simulink model "Comprobar_Posicion_PID_ISA"  (R2021b)
settings: Solver=ode45  StartTime=0.0  StopTime=100  RelTol=1e-3  EnableMultiTasking=on
undefined symbols (not defined in the file or in its folder): airspeed_0, alpha_0, altitude_0, beta_0, deflect_sat, Earth, euler_0, h0, JSBSim, local_V_0, mTotal, Pos_0, pqr_0, r_MotorLeft, r_MotorRight, theta_0, Vel_0, VTOL_FW, WGS84
libraries: simulink_need_slupdate x5, aerolibfltsims x4, sharedutil x3, sharedtransform x2, aerolibtransform2 x1, aerolibutil x1
(part 1 of 2)
settings Model: Creator=Fede Paredes  LastModifiedBy=Jose Luis Musoles
settings SolverCC: AlgebraicLoopSolver=TrustRegion
settings DataIOCC: LimitDataPoints=on  SaveFormat=Array  ReturnWorkspaceOutputs=off
settings OptimizationCC: LifeSpan=inf
settings DebuggingCC: UnderspecifiedInitializationDetection=Classic  MergeDetectMultiDrivingBlocksExec=none  SolverPrmCheckMsg=warning  StateNameClashWarn=warning  SFUnexpectedBacktrackingDiag=warning  SFNoUnconditionalDefaultTransitionDiag=warning  SFExecutionAtInitializationDiag=none  SFMachineParentedDataDiag=warning  ArithmeticOperatorsInVariantConditions=warning
settings HardwareCC: ProdBitPerPointer=32  ProdBitPerSizeT=32  ProdBitPerPtrDiffT=32  ProdLargestAtomicFloat=None  ProdIntDivRoundTo=Undefined  ProdEndianess=Unspecified  ProdWordSize=32  ProdHWDeviceType=32-bit Generic
settings ModelReferenceCC: PropagateSignalLabelsOutOfModel=off
settings SFSimCC: SimUseLocalCustomCode=off  CustomCodeUndefinedFunction=UseInterfaceOnly
settings RTWCC: RTWUseLocalCustomCode=off
settings CodeAppCC: StateflowObjectComments=on
settings GRTTargetCC: TargetLangStandard=C89/C90 (ANSI)
settings ConfigComp: CovMetricSettings=dw  CovSaveCumulativeToWorkspaceVar=on  CovSaveSingleToWorkspaceVar=on  CovExternalEMLEnable=off

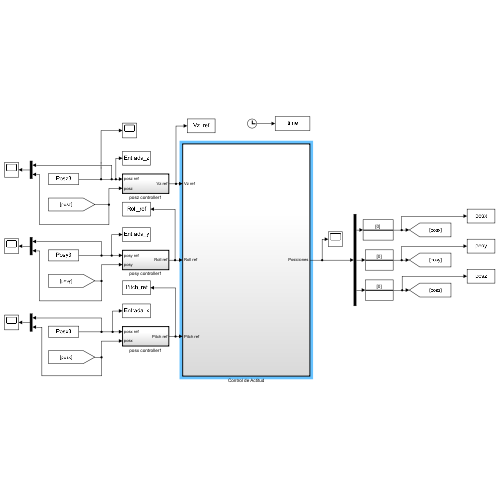
[thumbnail: Simulink's stored preview of the top-level diagram]
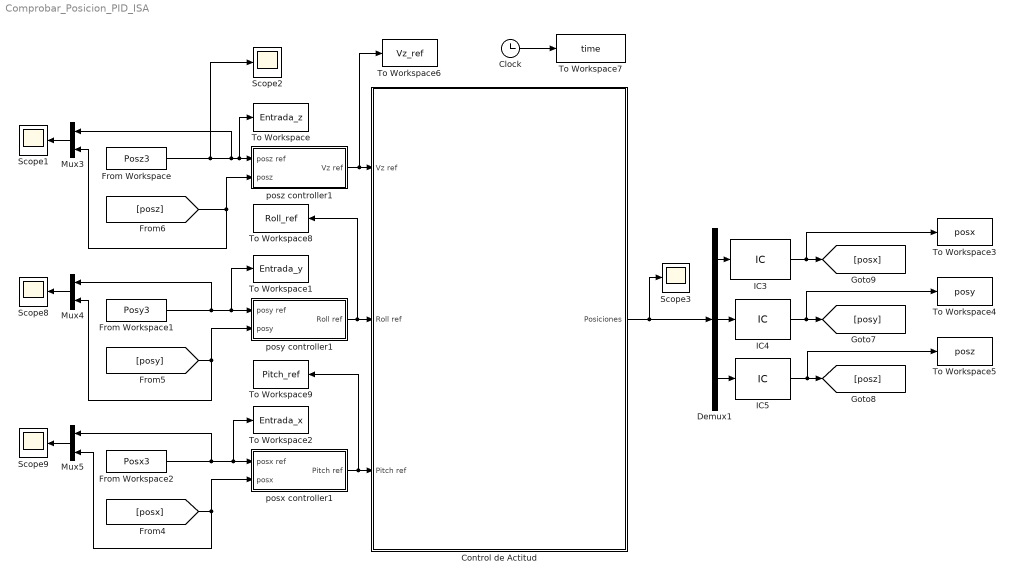
== system Comprobar_Posicion_PID_ISA ==
  Clock : Clock
  Control de Actitud : Subsystem  TreatAsAtomicUnit=on
  Demux1 : Demux  Outputs=3
  From Workspace : FromWorkspace  VariableName=Posz3
  From Workspace1 : FromWorkspace  VariableName=Posy3
  From Workspace2 : FromWorkspace  VariableName=Posx3
  IC3 : InitialCondition  Value=0
  IC4 : InitialCondition  Value=0
  IC5 : InitialCondition  Value=0
  Mux3 : Mux  Inputs=2
  Mux4 : Mux  Inputs=2
  Mux5 : Mux  Inputs=2
  Scope{1..3,8..9} (5 alike) : Scope
  To Workspace : ToWorkspace  VariableName=Entrada_z  SaveFormat=Timeseries  SampleTime=-1
  To Workspace1 : ToWorkspace  VariableName=Entrada_y  SaveFormat=Timeseries  SampleTime=-1
  To Workspace2 : ToWorkspace  VariableName=Entrada_x  SaveFormat=Timeseries  SampleTime=-1
  To Workspace3 : ToWorkspace  VariableName=posx  SaveFormat=Timeseries  SampleTime=-1
  To Workspace4 : ToWorkspace  VariableName=posy  SaveFormat=Timeseries  SampleTime=-1
  To Workspace5 : ToWorkspace  VariableName=posz  SaveFormat=Timeseries  SampleTime=-1
  To Workspace6 : ToWorkspace  VariableName=Vz_ref  SaveFormat=Timeseries  SampleTime=-1
  To Workspace7 : ToWorkspace  VariableName=time  SaveFormat=Timeseries  SampleTime=-1
  To Workspace8 : ToWorkspace  VariableName=Roll_ref  SaveFormat=Timeseries  SampleTime=-1
  To Workspace9 : ToWorkspace  VariableName=Pitch_ref  SaveFormat=Timeseries  SampleTime=-1
  posx controller1 : Subsystem  TreatAsAtomicUnit=on
  posy controller1 : Subsystem  TreatAsAtomicUnit=on
  posz controller1 : Subsystem  TreatAsAtomicUnit=on
  wires:
  Control de Actitud/1(Posiciones) -> Demux1/1, Scope3/1
  Demux1/1 -> IC3/1
  Demux1/2 -> IC4/1
  Demux1/3 -> IC5/1
  posy controller1/1(Roll ref) -> To Workspace8/1, Control de Actitud/2(Roll ref)
  posx controller1/1(Pitch ref) -> To Workspace9/1, Control de Actitud/3(Pitch ref)
  [posx] -> posx controller1/2(posx), Mux5/2
  [posz] -> posz controller1/2(posz), Mux3/2
  [posy] -> posy controller1/2(posy), Mux4/2
  Mux3/1 -> Scope1/1
  Mux4/1 -> Scope8/1
  Mux5/1 -> Scope9/1
  From Workspace1/1 -> To Workspace1/1, posy controller1/1(posy ref), Mux4/1
  From Workspace2/1 -> To Workspace2/1, posx controller1/1(posx ref), Mux5/1
  From Workspace/1 -> Scope2/1, Mux3/1, To Workspace/1, posz controller1/1(posz ref)
  Clock/1 -> To Workspace7/1
  posz controller1/1(Vz ref) -> To Workspace6/1, Control de Actitud/1(Vz ref)
  IC5/1 -> To Workspace5/1, [posz]
  IC3/1 -> To Workspace3/1, [posx]
  IC4/1 -> To Workspace4/1, [posy]

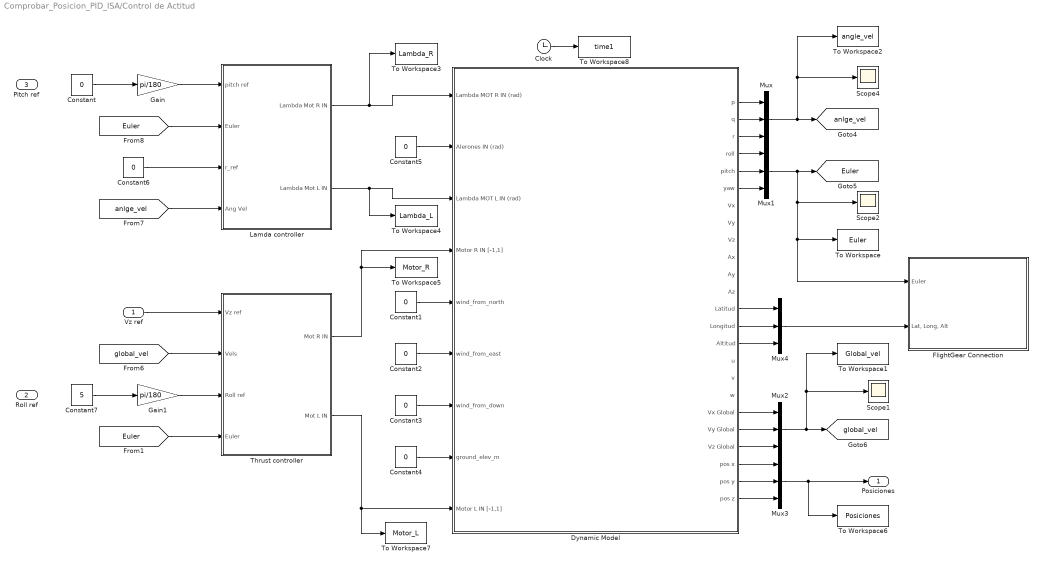
== system Comprobar_Posicion_PID_ISA/Control de Actitud ==
  Vz ref : Inport
  Roll ref : Inport  Port=2
  Pitch ref : Inport  Port=3
  Clock : Clock
  Constant{,1..6} (7 alike) : Constant  Value=0
  Constant7 : Constant  Value=5
  Dynamic Model : Subsystem  TreatAsAtomicUnit=on
  FlightGear Connection : Subsystem  TreatAsAtomicUnit=on
  Gain : Gain  Gain=pi/180
  Gain1 : Gain  Gain=pi/180
  Lamda controller : Subsystem
  Mux{,1..4} (5 alike) : Mux  Inputs=3
  Scope1 : Scope
  Scope2 : Scope
  Scope4 : Scope
  Thrust controller : Subsystem
  To Workspace : ToWorkspace  VariableName=Euler  SaveFormat=Timeseries  SampleTime=-1
  To Workspace1 : ToWorkspace  VariableName=Global_vel  SaveFormat=Timeseries  SampleTime=-1
  To Workspace2 : ToWorkspace  VariableName=angle_vel  SaveFormat=Timeseries  SampleTime=-1
  To Workspace3 : ToWorkspace  VariableName=Lambda_R  SaveFormat=Timeseries  SampleTime=-1
  To Workspace4 : ToWorkspace  VariableName=Lambda_L  SaveFormat=Timeseries  SampleTime=-1
  To Workspace5 : ToWorkspace  VariableName=Motor_R  SaveFormat=Timeseries  SampleTime=-1
  To Workspace6 : ToWorkspace  VariableName=Posiciones  SaveFormat=Timeseries  SampleTime=-1
  To Workspace7 : ToWorkspace  VariableName=Motor_L  SaveFormat=Timeseries  SampleTime=-1
  To Workspace8 : ToWorkspace  VariableName=time1  SaveFormat=Timeseries  SampleTime=-1
  Posiciones : Outport
  tag scope: Euler=global, anlge_vel=global, global_vel=global
  wires:
  Dynamic Model/1(p) -> Mux/1
  Dynamic Model/3(r) -> Mux/3
  Mux/1 -> To Workspace2/1, Scope4/1, [anlge_vel]
  Dynamic Model/4(roll) -> Mux1/1
  Dynamic Model/6(yaw) -> Mux1/3
  Mux1/1 -> FlightGear Connection/1("Euler "), To Workspace/1, Scope2/1, [Euler]
  Dynamic Model/2(q) -> Mux/2
  Dynamic Model/5(pitch) -> Mux1/2
  Mux2/1 -> Scope1/1, To Workspace1/1, [global_vel]
  [global_vel] -> Thrust controller/2(Vels)
  Thrust controller/1(Mot R IN) -> To Workspace5/1, Dynamic Model/4(Motor R IN [-1,1])
  Thrust controller/2(Mot L IN) -> To Workspace7/1, Dynamic Model/9(Motor L IN [-1,1])
  [Euler] -> Thrust controller/4(Euler)
  [Euler] -> Lamda controller/2(Euler)
  [anlge_vel] -> Lamda controller/4(Ang Vel)
  Lamda controller/1(Lambda Mot R IN) -> To Workspace3/1, Dynamic Model/1(Lambda MOT R IN (rad))
  Lamda controller/2(Lambda Mot L IN) -> To Workspace4/1, Dynamic Model/3(" Lambda MOT L IN (rad)")
  Constant5/1 -> Dynamic Model/2(Alerones IN (rad))
  Vz ref/1 -> Thrust controller/1(Vz ref)
  Constant6/1 -> Lamda controller/3(r_ref)
  Mux3/1 -> Posiciones/1, To Workspace6/1
  Constant1/1 -> Dynamic Model/5(wind_from_north)
  Constant2/1 -> Dynamic Model/6(wind_from_east)
  Constant3/1 -> Dynamic Model/7(wind_from_down)
  Constant4/1 -> Dynamic Model/8(ground_elev_m)
  Dynamic Model/22(pos x) -> Mux3/1
  Dynamic Model/23(pos y) -> Mux3/2
  Dynamic Model/24(pos z) -> Mux3/3
  Dynamic Model/19(Vx Global) -> Mux2/1
  Dynamic Model/20(Vy Global) -> Mux2/2
  Dynamic Model/21(Vz Global) -> Mux2/3
  Clock/1 -> To Workspace8/1
  Dynamic Model/13(Latitud) -> Mux4/1
  Dynamic Model/14(Longitud) -> Mux4/2
  Dynamic Model/15(Altitud) -> Mux4/3
  Mux4/1 -> FlightGear Connection/2("Lat, Long, Alt ")
  Constant/1 -> Gain/1
  Gain/1 -> Lamda controller/1(pitch ref)
  Constant7/1 -> Gain1/1
  Gain1/1 -> Thrust controller/3(Roll ref)

== system Comprobar_Posicion_PID_ISA/posx controller1 ==
  posx ref : Inport
  posx : Inport  Port=2
  Constant : Constant  Value=0
  PID ISA : Subsystem  mask{kc=-0.5363, Ti=17.0146, Td=0.8299}
  Rate Transition : RateTransition  OutPortSampleTime=2e-2
  Rate Transition1 : RateTransition  OutPortSampleTime=2e-2
  Scope4 : Scope
  Pitch ref : Outport
  wires:
  posx ref/1 -> Rate Transition/1
  posx/1 -> Rate Transition1/1
  Constant/1 -> PID ISA/3(u0)
  Rate Transition/1 -> PID ISA/1(Reference)
  Rate Transition1/1 -> PID ISA/2(Vc)
  PID ISA/1(Vm) -> Scope4/1, Pitch ref/1

== system Comprobar_Posicion_PID_ISA/posy controller1 ==
  posy ref : Inport
  posy : Inport  Port=2
  Constant : Constant  Value=0
  PID ISA : Subsystem  mask{kc=0.5691, Ti=16.6404, Td=0.9487}
  Rate Transition : RateTransition  OutPortSampleTime=2e-2
  Rate Transition1 : RateTransition  OutPortSampleTime=2e-2
  Scope4 : Scope
  Roll ref : Outport
  wires:
  Constant/1 -> PID ISA/3(u0)
  posy ref/1 -> Rate Transition/1
  Rate Transition/1 -> PID ISA/1(Reference)
  posy/1 -> Rate Transition1/1
  Rate Transition1/1 -> PID ISA/2(Vc)
  PID ISA/1(Vm) -> Scope4/1, Roll ref/1

== system Comprobar_Posicion_PID_ISA/posz controller1 ==
  note: Se ha modificado la derivada
  posz ref : Inport
  posz : Inport  Port=2
  Constant : Constant  Value=0
  PID ISA : Subsystem  mask{kc=0.9270, Ti=10.0761, Td=0.4708}
  Rate Transition : RateTransition  OutPortSampleTime=2e-2
  Rate Transition1 : RateTransition  OutPortSampleTime=2e-2
  Scope4 : Scope
  Vz ref : Outport
  wires:
  Constant/1 -> PID ISA/3(u0)
  posz ref/1 -> Rate Transition/1
  Rate Transition/1 -> PID ISA/1(Reference)
  posz/1 -> Rate Transition1/1
  Rate Transition1/1 -> PID ISA/2(Vc)
  PID ISA/1(Vm) -> Scope4/1, Vz ref/1

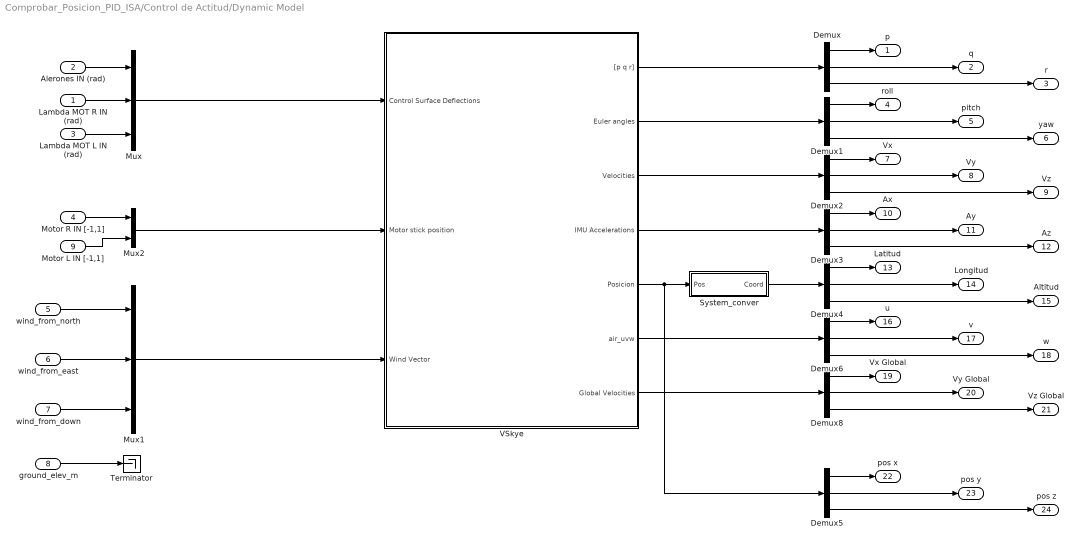
== system Comprobar_Posicion_PID_ISA/Control de Actitud/Dynamic Model ==
  Lambda MOT R IN (rad) : Inport
  Alerones IN (rad) : Inport  Port=2
  " Lambda MOT L IN (rad)" : Inport  Port=3
  Motor R IN [-1,1] : Inport  Port=4
  wind_from_north : Inport  Port=5
  wind_from_east : Inport  Port=6
  wind_from_down : Inport  Port=7
  ground_elev_m : Inport  Port=8
  Motor L IN [-1,1] : Inport  Port=9
  Demux{,1..6,8} (8 alike) : Demux  Outputs=3
  Mux : Mux  Inputs=3
  Mux1 : Mux  Inputs=3
  Mux2 : Mux  Inputs=2
  System_conver : Subsystem
  Terminator : Terminator
  VSkye : Subsystem
  p : Outport
  q : Outport  Port=2
  r : Outport  Port=3
  roll : Outport  Port=4
  pitch : Outport  Port=5
  yaw : Outport  Port=6
  Vx : Outport  Port=7
  Vy : Outport  Port=8
  Vz : Outport  Port=9
  Ax : Outport  Port=10
  Ay : Outport  Port=11
  Az : Outport  Port=12
  Latitud : Outport  Port=13
  Longitud : Outport  Port=14
  Altitud : Outport  Port=15
  u : Outport  Port=16
  v : Outport  Port=17
  w : Outport  Port=18
  Vx Global : Outport  Port=19
  Vy Global : Outport  Port=20
  Vz Global : Outport  Port=21
  pos x : Outport  Port=22
  pos y : Outport  Port=23
  pos z : Outport  Port=24
  wires:
  VSkye/2(Euler angles) -> Demux1/1
  VSkye/3(Velocities) -> Demux2/1
  Mux1/1 -> VSkye/3(Wind Vector)
  VSkye/5(Posicion) -> Demux5/1, System_conver/1(Pos)
  Mux/1 -> VSkye/1(Control Surface Deflections)
  VSkye/4("IMU Accelerations ") -> Demux3/1
  VSkye/1("[p q r]") -> Demux/1
  Alerones IN (rad)/1 -> Mux/1
  Lambda MOT R IN (rad)/1 -> Mux/2
  " Lambda MOT L IN (rad)"/1 -> Mux/3
  Demux/1 -> p/1
  Demux/2 -> q/1
  Demux/3 -> r/1
  Demux1/1 -> roll/1
  Demux1/2 -> pitch/1
  Demux1/3 -> yaw/1
  Demux2/1 -> Vx/1
  Demux2/2 -> Vy/1
  Demux2/3 -> Vz/1
  Demux3/1 -> Ax/1
  Demux3/2 -> Ay/1
  Demux3/3 -> Az/1
  Demux4/1 -> Latitud/1
  Demux4/2 -> Longitud/1
  Demux4/3 -> Altitud/1
  Demux6/1 -> u/1
  Demux6/2 -> v/1
  Demux6/3 -> w/1
  Demux5/1 -> pos x/1
  Demux5/2 -> pos y/1
  Demux5/3 -> pos z/1
  VSkye/6(air_uvw) -> Demux6/1
  System_conver/1(Coord) -> Demux4/1
  wind_from_north/1 -> Mux1/1
  wind_from_east/1 -> Mux1/2
  wind_from_down/1 -> Mux1/3
  Motor R IN [-1,1]/1 -> Mux2/1
  Mux2/1 -> VSkye/2(Motor stick position)
  Motor L IN [-1,1]/1 -> Mux2/2
  ground_elev_m/1 -> Terminator/1
  Demux8/1 -> Vx Global/1
  Demux8/2 -> Vy Global/1
  Demux8/3 -> Vz Global/1
  VSkye/7(Global Velocities) -> Demux8/1

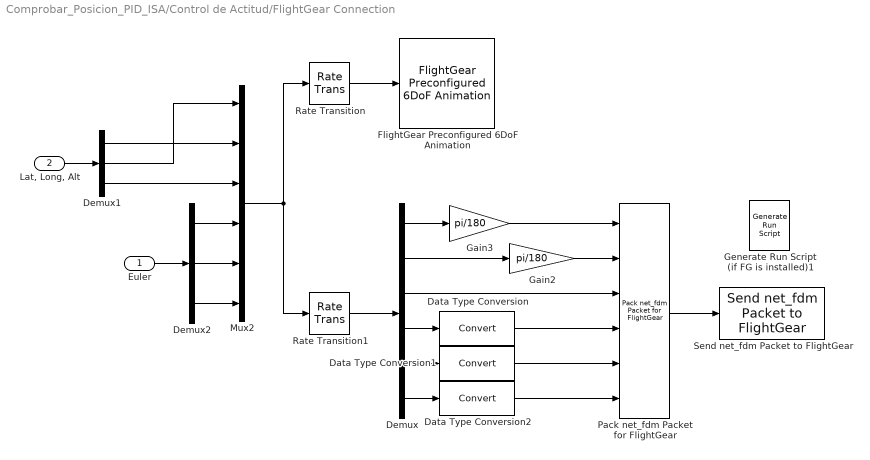
== system Comprobar_Posicion_PID_ISA/Control de Actitud/FlightGear Connection ==
  "Euler " : Inport
  "Lat, Long, Alt " : Inport  Port=2
  Data Type Conversion : DataTypeConversion  SampleTime=0.01
  Data Type Conversion1 : DataTypeConversion  SampleTime=0.01
  Data Type Conversion2 : DataTypeConversion  SampleTime=0.01
  Demux : Demux  Outputs=6
  Demux1 : Demux  Outputs=3
  Demux2 : Demux  Outputs=3
  FlightGear Preconfigured 6DoF Animation : aerolibfltsims/FlightGear Preconfigured 6DoF Animation  xFlightGearVersion=v2.6  DestinationIpAddress=127.0.0.1  DestinationPort=5502  SampleTime=0.01  packetVersion=24
  Gain2 : Gain  Gain=pi/180
  Gain3 : Gain  Gain=pi/180
  Generate Run Script (if FG is installed)1 : aerolibfltsims/Generate Run Script  Architecture=Default  dataFlow=Send  GeometryModelName=VTOL_FW-JSBSim  AirportId=KSFO  RunwayId=10L  InitialAltitude=7224  InitialHeading=113  OffsetDistance=4.72  OffsetAzimuth=0  InstallScenery=off  DisableShaders=off  OriginAddress=127.0.0.1  DestinationPort=5502  OriginPort=5505  LocalAddress=127.0.0.1  OutputFileName=FW_Simulink26.bat  FlightGearBaseDirectory=C:\Program Files\FlightGear2.6
  Mux2 : Mux  Inputs=6
  Pack net_fdm Packet for FlightGear : aerolibfltsims/Pack net_fdm Packet for FlightGear  FlightGearVersion=v2.6  ShowPositionAttitudeInputs=on  ShowVelocityAccelerationInputs=off  ShowControlSurfacePositionInputs=off  ShowEngineFuelInputs=off  ShowLandingGearInputs=off  ShowEnvironmentInputs=off  SampleTime=0.01  packetVersion=24
      settings: SourceProductBaseCode=AE
  Rate Transition : RateTransition  InitialCondition=[0,0,0,pi,0,0]
  Rate Transition1 : RateTransition  InitialCondition=[0,0,0,0,0,0]
  Send net_fdm Packet to FlightGear : aerolibfltsims/Send net_fdm Packet to FlightGear  DestinationIpAddress=127.0.0.1  DestinationPort=5502  LocalIpPort=-1  varLen=off  SampleTime=0.01
      settings: SourceProductBaseCode=AE
  wires:
  Demux2/1 -> Mux2/4
  Demux2/2 -> Mux2/5
  Demux2/3 -> Mux2/6
  Demux/1 -> Gain3/1
  Demux/2 -> Gain2/1
  Demux/3 -> Pack net_fdm Packet for FlightGear/3
  Pack net_fdm Packet for FlightGear/1 -> Send net_fdm Packet to FlightGear/1
  "Euler "/1 -> Demux2/1
  "Lat, Long, Alt "/1 -> Demux1/1
  Rate Transition/1 -> FlightGear Preconfigured 6DoF Animation/1
  Rate Transition1/1 -> Demux/1
  Demux/6 -> Data Type Conversion2/1
  Demux/5 -> Data Type Conversion1/1
  Demux/4 -> Data Type Conversion/1
  Data Type Conversion/1 -> Pack net_fdm Packet for FlightGear/4
  Data Type Conversion1/1 -> Pack net_fdm Packet for FlightGear/5
  Data Type Conversion2/1 -> Pack net_fdm Packet for FlightGear/6
  Demux1/3 -> Mux2/3
  Mux2/1 -> Rate Transition1/1, Rate Transition/1
  Gain3/1 -> Pack net_fdm Packet for FlightGear/1
  Gain2/1 -> Pack net_fdm Packet for FlightGear/2
  Demux1/1 -> Mux2/2
  Demux1/2 -> Mux2/1

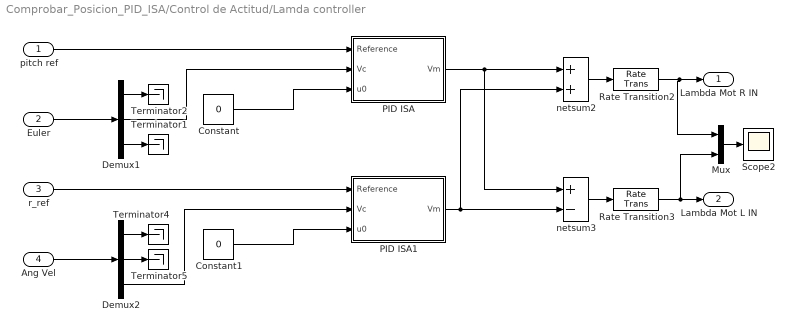
== system Comprobar_Posicion_PID_ISA/Control de Actitud/Lamda controller ==
  pitch ref : Inport
  Euler : Inport  Port=2
  r_ref : Inport  Port=3
  Ang Vel : Inport  Port=4
  Constant : Constant  Value=0
  Constant1 : Constant  Value=0
  Demux1 : Demux  Outputs=3
  Demux2 : Demux  Outputs=3
  Mux : Mux  Inputs=2
  PID ISA : Subsystem  mask{kc=0.549, Ti=0.450, Td=0.111}
  PID ISA1 : Subsystem  mask{kc=0.2421, Ti=6.3879, Td=0.0264}
  Rate Transition2 : RateTransition  OutPortSampleTime=1e-2
  Rate Transition3 : RateTransition  OutPortSampleTime=1e-2
  Scope2 : Scope
  Terminator{1..2,4..5} (4 alike) : Terminator
  netsum2 : Sum  Inputs=2  InputSameDT=on  SaturateOnIntegerOverflow=on  OutDataTypeStr=Inherit: Same as first input
  netsum3 : Sum  Inputs=+-  InputSameDT=on  SaturateOnIntegerOverflow=on  OutDataTypeStr=Inherit: Same as first input
  Lambda Mot R IN : Outport
  Lambda Mot L IN : Outport  Port=2
  wires:
  Demux1/1 -> Terminator2/1
  Euler/1 -> Demux1/1
  Demux1/3 -> Terminator1/1
  Demux2/1 -> Terminator4/1
  Ang Vel/1 -> Demux2/1
  Demux2/2 -> Terminator5/1
  PID ISA/1(Vm) -> netsum3/1, netsum2/1
  PID ISA1/1(Vm) -> netsum2/2, netsum3/2
  netsum2/1 -> Rate Transition2/1
  netsum3/1 -> Rate Transition3/1
  pitch ref/1 -> PID ISA/1(Reference)
  r_ref/1 -> PID ISA1/1(Reference)
  Demux1/2 -> PID ISA/2(Vc)
  Constant/1 -> PID ISA/3(u0)
  Demux2/3 -> PID ISA1/2(Vc)
  Constant1/1 -> PID ISA1/3(u0)
  Rate Transition2/1 -> Mux/1, Lambda Mot R IN/1
  Rate Transition3/1 -> Mux/2, Lambda Mot L IN/1
  Mux/1 -> Scope2/1

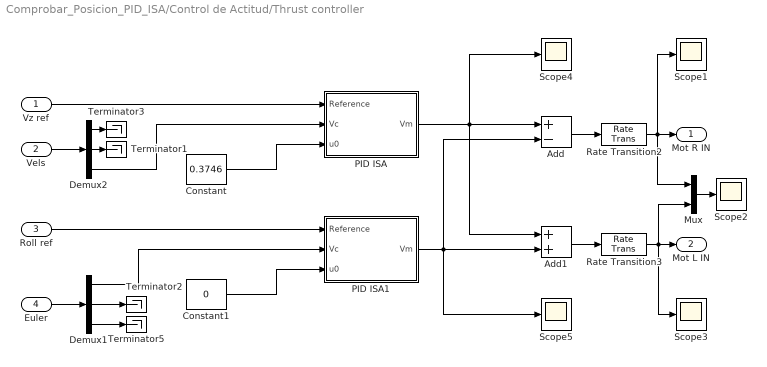
== system Comprobar_Posicion_PID_ISA/Control de Actitud/Thrust controller ==
  Vz ref : Inport
  Vels : Inport  Port=2
  Roll ref : Inport  Port=3
  Euler : Inport  Port=4
  Add : Sum  Inputs=+-
  Add1 : Sum
  Constant : Constant  Value=0.3746
  Constant1 : Constant  Value=0
  Demux1 : Demux  Outputs=3
  Demux2 : Demux  Outputs=3
  Mux : Mux  Inputs=2
  PID ISA : Subsystem  mask{kc=-0.42, Ti=11.3514, Td=0.0471}
  PID ISA1 : Subsystem  mask{kc=0.8757, Ti=0.4816, Td=0.1199}
  Rate Transition2 : RateTransition  OutPortSampleTime=1e-2
  Rate Transition3 : RateTransition  OutPortSampleTime=1e-2
  Scope{1..5} (5 alike) : Scope
  Terminator{1..3,5} (4 alike) : Terminator
  Mot R IN : Outport
  Mot L IN : Outport  Port=2
  wires:
  Mux/1 -> Scope2/1
  Constant1/1 -> PID ISA1/3(u0)
  Demux1/1 -> PID ISA1/2(Vc)
  Constant/1 -> PID ISA/3(u0)
  Demux2/3 -> PID ISA/2(Vc)
  Rate Transition3/1 -> Scope3/1, Mot L IN/1, Mux/2
  Rate Transition2/1 -> Mux/1, Scope1/1, Mot R IN/1
  Roll ref/1 -> PID ISA1/1(Reference)
  Vz ref/1 -> PID ISA/1(Reference)
  PID ISA1/1(Vm) -> Scope5/1, Add/2, Add1/2
  Add1/1 -> Rate Transition3/1
  PID ISA/1(Vm) -> Scope4/1, Add/1, Add1/1
  Add/1 -> Rate Transition2/1
  Demux1/3 -> Terminator5/1
  Demux1/2 -> Terminator2/1
  Euler/1 -> Demux1/1
  Vels/1 -> Demux2/1
  Demux2/2 -> Terminator1/1
  Demux2/1 -> Terminator3/1

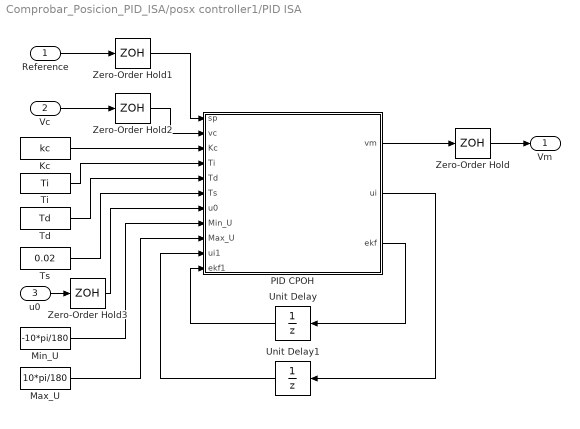
== system Comprobar_Posicion_PID_ISA/posx controller1/PID ISA ==
  Reference : Inport
  Vc : Inport  Port=2
  u0 : Inport  Port=3
  Kc : Constant  Value=kc
  Max_U : Constant  Value=10*pi/180
  Min_U : Constant  Value=-10*pi/180
  PID CPOH : MATLAB Function  TreatAsAtomicUnit=on
  Td : Constant  Value=Td
  Ti : Constant  Value=Ti
  Ts : Constant  Value=0.02
  Unit Delay : UnitDelay  SampleTime=0.02  HasFrameUpgradeWarning=on
  Unit Delay1 : UnitDelay  SampleTime=0.02  HasFrameUpgradeWarning=on
  Zero-Order Hold : ZeroOrderHold  SampleTime=0.02
  Zero-Order Hold1 : ZeroOrderHold  SampleTime=0.02
  Zero-Order Hold2 : ZeroOrderHold  SampleTime=0.02
  Zero-Order Hold3 : ZeroOrderHold  SampleTime=0.04
  Vm : Outport
  wires:
  Kc/1 -> PID CPOH/3(Kc)
  Ti/1 -> PID CPOH/4(Ti)
  Td/1 -> PID CPOH/5(Td)
  Ts/1 -> PID CPOH/6(Ts)
  u0/1 -> Zero-Order Hold3/1
  Min_U/1 -> PID CPOH/8(Min_U)
  Max_U/1 -> PID CPOH/9(Max_U)
  Unit Delay/1 -> PID CPOH/11(ekf1)
  PID CPOH/3(ekf) -> Unit Delay/1
  Unit Delay1/1 -> PID CPOH/10(ui1)
  PID CPOH/2(ui) -> Unit Delay1/1
  Reference/1 -> Zero-Order Hold1/1
  Vc/1 -> Zero-Order Hold2/1
  PID CPOH/1(vm) -> Zero-Order Hold/1
  Zero-Order Hold/1 -> Vm/1
  Zero-Order Hold1/1 -> PID CPOH/1(sp)
  Zero-Order Hold3/1 -> PID CPOH/7(u0)
  Zero-Order Hold2/1 -> PID CPOH/2(vc)

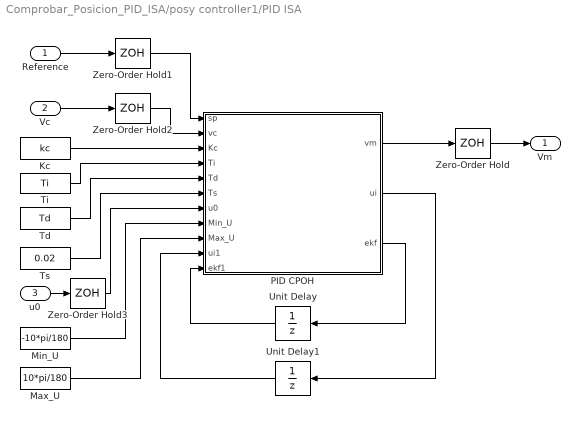
== system Comprobar_Posicion_PID_ISA/posy controller1/PID ISA ==
  Reference : Inport
  Vc : Inport  Port=2
  u0 : Inport  Port=3
  Kc : Constant  Value=kc
  Max_U : Constant  Value=10*pi/180
  Min_U : Constant  Value=-10*pi/180
  PID CPOH : MATLAB Function  TreatAsAtomicUnit=on
  Td : Constant  Value=Td
  Ti : Constant  Value=Ti
  Ts : Constant  Value=0.02
  Unit Delay : UnitDelay  SampleTime=0.02  HasFrameUpgradeWarning=on
  Unit Delay1 : UnitDelay  SampleTime=0.02  HasFrameUpgradeWarning=on
  Zero-Order Hold : ZeroOrderHold  SampleTime=0.02
  Zero-Order Hold1 : ZeroOrderHold  SampleTime=0.02
  Zero-Order Hold2 : ZeroOrderHold  SampleTime=0.02
  Zero-Order Hold3 : ZeroOrderHold  SampleTime=0.04
  Vm : Outport
  wires:
  Kc/1 -> PID CPOH/3(Kc)
  Ti/1 -> PID CPOH/4(Ti)
  Td/1 -> PID CPOH/5(Td)
  Ts/1 -> PID CPOH/6(Ts)
  u0/1 -> Zero-Order Hold3/1
  Min_U/1 -> PID CPOH/8(Min_U)
  Max_U/1 -> PID CPOH/9(Max_U)
  Unit Delay/1 -> PID CPOH/11(ekf1)
  PID CPOH/3(ekf) -> Unit Delay/1
  Unit Delay1/1 -> PID CPOH/10(ui1)
  PID CPOH/2(ui) -> Unit Delay1/1
  Reference/1 -> Zero-Order Hold1/1
  Vc/1 -> Zero-Order Hold2/1
  PID CPOH/1(vm) -> Zero-Order Hold/1
  Zero-Order Hold/1 -> Vm/1
  Zero-Order Hold1/1 -> PID CPOH/1(sp)
  Zero-Order Hold3/1 -> PID CPOH/7(u0)
  Zero-Order Hold2/1 -> PID CPOH/2(vc)

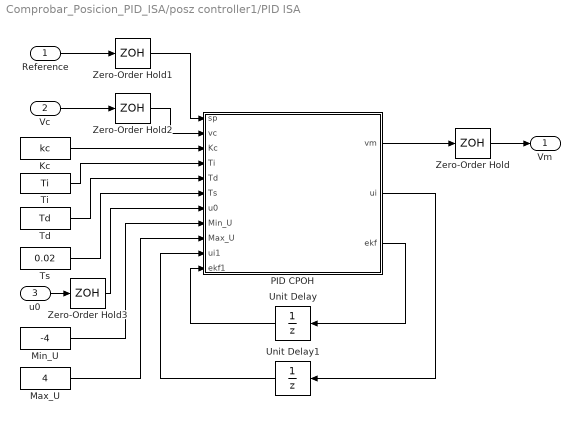
== system Comprobar_Posicion_PID_ISA/posz controller1/PID ISA ==
  Reference : Inport
  Vc : Inport  Port=2
  u0 : Inport  Port=3
  Kc : Constant  Value=kc
  Max_U : Constant  Value=4
  Min_U : Constant  Value=-4
  PID CPOH : MATLAB Function  TreatAsAtomicUnit=on
  Td : Constant  Value=Td
  Ti : Constant  Value=Ti
  Ts : Constant  Value=0.02
  Unit Delay : UnitDelay  SampleTime=0.02  HasFrameUpgradeWarning=on
  Unit Delay1 : UnitDelay  SampleTime=0.02  HasFrameUpgradeWarning=on
  Zero-Order Hold : ZeroOrderHold  SampleTime=0.02
  Zero-Order Hold1 : ZeroOrderHold  SampleTime=0.02
  Zero-Order Hold2 : ZeroOrderHold  SampleTime=0.02
  Zero-Order Hold3 : ZeroOrderHold  SampleTime=0.04
  Vm : Outport
  wires:
  Kc/1 -> PID CPOH/3(Kc)
  Ti/1 -> PID CPOH/4(Ti)
  Td/1 -> PID CPOH/5(Td)
  Ts/1 -> PID CPOH/6(Ts)
  u0/1 -> Zero-Order Hold3/1
  Min_U/1 -> PID CPOH/8(Min_U)
  Max_U/1 -> PID CPOH/9(Max_U)
  Unit Delay/1 -> PID CPOH/11(ekf1)
  PID CPOH/3(ekf) -> Unit Delay/1
  Unit Delay1/1 -> PID CPOH/10(ui1)
  PID CPOH/2(ui) -> Unit Delay1/1
  Reference/1 -> Zero-Order Hold1/1
  Vc/1 -> Zero-Order Hold2/1
  PID CPOH/1(vm) -> Zero-Order Hold/1
  Zero-Order Hold/1 -> Vm/1
  Zero-Order Hold1/1 -> PID CPOH/1(sp)
  Zero-Order Hold3/1 -> PID CPOH/7(u0)
  Zero-Order Hold2/1 -> PID CPOH/2(vc)

== system Comprobar_Posicion_PID_ISA/Control de Actitud/Dynamic Model/System_conver ==
  note: Coordenadas aeropuerto Valencia 39.491424,-0.486812
  note: Coordenadas iniciales aeroclub Cheste
  Pos : Inport
  Flat_Earth_to_LLA : aerolibtransform2/Flat Earth to LLA  units=Metric (MKS)  ptype=Earth (WGS84)  F=1/298.257223563  R=6378137  refPosPort=off  LL0=[39.4975172153840717,-0.626435279846191406]  psi=0
  Mux : Mux  Inputs=2
  h0 : Constant  Value=0
  Coord : Outport
  wires:
  Pos/1 -> Flat_Earth_to_LLA/1
  h0/1 -> Flat_Earth_to_LLA/2
  Flat_Earth_to_LLA/2 -> Mux/2
  Flat_Earth_to_LLA/1 -> Mux/1
  Mux/1 -> Coord/1

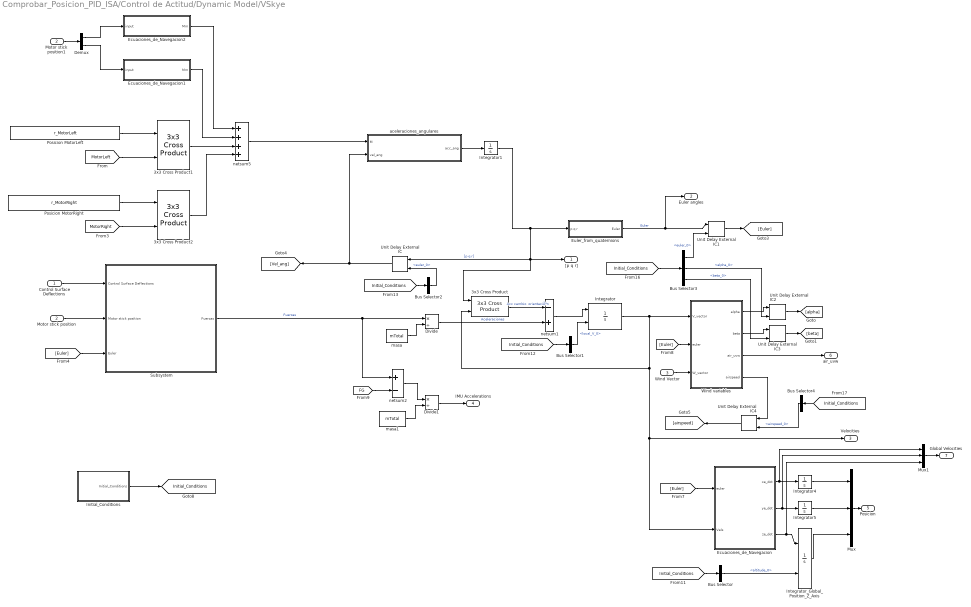
== system Comprobar_Posicion_PID_ISA/Control de Actitud/Dynamic Model/VSkye ==
  Control Surface Deflections : Inport  PortDimensions=3
  Motor stick position : Inport  Port=2  PortDimensions=2
  Wind Vector : Inport  Port=3
  3x3 Cross Product : sharedutil/3x3 Cross Product  aMode=aMode
      settings: SourceProductBaseCode=AE,PW,DR,MT,UV,VE
  3x3 Cross Product1 : sharedutil/3x3 Cross Product  aMode=aMode
      settings: SourceProductBaseCode=AE,PW,DR,MT,UV,VE
  3x3 Cross Product2 : sharedutil/3x3 Cross Product  aMode=aMode
      settings: SourceProductBaseCode=AE,PW,DR,MT,UV,VE
  Bus Selector : BusSelector  OutputSignals=altitude_0
  Bus Selector1 : BusSelector  OutputSignals=local_V_0
  Bus Selector2 : BusSelector  OutputSignals=euler_0
  Bus Selector3 : BusSelector  OutputSignals=euler_0,alpha_0,beta_0
  Bus Selector4 : BusSelector  OutputSignals=airspeed_0
  Demux : Demux  Outputs=2
  Divide : Product  Inputs=*/
  Divide1 : Product  Inputs=*/
  Ecuaciones_de_Navegacion : MATLAB Function  TreatAsAtomicUnit=on
  Ecuaciones_de_Navegacion1 : MATLAB Function  TreatAsAtomicUnit=on
  Ecuaciones_de_Navegacion2 : MATLAB Function  TreatAsAtomicUnit=on
  Euler_from_quaternions : Subsystem
  Initial_Conditions : Subsystem
  Integrator : Integrator  InitialConditionSource=external
  Integrator1 : Integrator  InitialCondition=[0 0 0]
  Integrator4 : Integrator
  Integrator5 : Integrator
  Integrator_Global_Position_Z_Axis : Integrator  InitialConditionSource=external  UpperSaturationLimit=0
  Motor stick position1 : InportShadow  Port=2  PortDimensions=2
  Mux : Mux  Inputs=3
  Mux1 : Mux  Inputs=3
  Posicion MotorLeft : Constant  Value=r_MotorLeft
  Posicion MotorRight : Constant  Value=r_MotorRight
  Subsystem : Subsystem
  Unit Delay External IC{,1..4} (5 alike) : simulink_need_slupdate/Unit Delay External IC  tsamp=-1
      settings: SourceProductBaseCode=SL
  Wind variables : MATLAB Function  TreatAsAtomicUnit=on
  aceleraciones_angulares : MATLAB Function  TreatAsAtomicUnit=on
  masa : Constant  Value=mTotal
  masa1 : Constant  Value=mTotal
  netsum1 : Sum  Inputs=-+  InputSameDT=on  SaturateOnIntegerOverflow=on  OutDataTypeStr=Inherit: Same as first input
  netsum2 : Sum  Inputs=+-  InputSameDT=on  SaturateOnIntegerOverflow=on  OutDataTypeStr=Inherit: Same as first input
  netsum5 : Sum  Inputs=4  InputSameDT=on  SaturateOnIntegerOverflow=on  OutDataTypeStr=Inherit: Same as first input
  "[p q r]" : Outport
  Euler angles : Outport  Port=2
  Velocities : Outport  Port=3
  "IMU Accelerations " : Outport  Port=4
  Posicion : Outport  Port=5
  air_uvw : Outport  Port=6
  Global Velocities : Outport  Port=7
  tag scope: Initial_Conditions=global
  wires:
  Subsystem/1(Fuerzas) -> Divide/1, netsum2/1  "Fuerzas"
  Euler_from_quaternions/1(Euler) -> Euler angles/1, Unit Delay External IC1/1  "Euler"
  Unit Delay External IC1/1 -> [Euler]
  Wind variables/1(alpha) -> Unit Delay External IC2/1
  Wind variables/2(beta) -> Unit Delay External IC3/1
  Unit Delay External IC/1 -> [Vel_ang], aceleraciones_angulares/2(vel_ang)
  [Euler] -> Ecuaciones_de_Navegacion/1(euler)
  Ecuaciones_de_Navegacion/3(ze_dot) -> Mux1/3, Integrator_Global_Position_Z_Axis/1
  Ecuaciones_de_Navegacion/1(xe_dot) -> Mux1/1, Integrator4/1
  Ecuaciones_de_Navegacion/2(ye_dot) -> Mux1/2, Integrator5/1
  Unit Delay External IC3/1 -> [beta]
  masa/1 -> Divide/2
  Unit Delay External IC2/1 -> [alpha]
  Wind Vector/1 -> Wind variables/3(W_vector)
  [Euler] -> Wind variables/2(euler)
  Wind variables/4(airspeed) -> Unit Delay External IC4/1
  Unit Delay External IC4/1 -> [airspeed]
  aceleraciones_angulares/1(acc_ang) -> Integrator1/1
  netsum2/1 -> Divide1/1
  [FG] -> netsum2/2
  masa1/1 -> Divide1/2
  Divide1/1 -> "IMU Accelerations "/1
  Integrator4/1 -> Mux/1
  Integrator5/1 -> Mux/2
  Mux/1 -> Posicion/1
  Wind variables/3(air_uvw) -> air_uvw/1
  Integrator1/1 -> "[p q r]"/1, 3x3 Cross Product/1, Unit Delay External IC/1, Euler_from_quaternions/1(p q r)  "[p q r]"
  3x3 Cross Product/1 -> netsum1/1  "Acc cambio  orientaciÃ³n"
  netsum1/1 -> Integrator/1
  Divide/1 -> netsum1/2  "Aceleraciones"
  Integrator_Global_Position_Z_Axis/1 -> Mux/3
  Integrator/1 -> 3x3 Cross Product/2, Ecuaciones_de_Navegacion/2(Vels), Velocities/1, Wind variables/1(V_vector)
  Initial_Conditions/1(Initial_Conditions) -> [Initial_Conditions]
  [Initial_Conditions] -> Bus Selector/1
  Bus Selector/1 -> Integrator_Global_Position_Z_Axis/2  "<altitude_0>"
  [Initial_Conditions] -> Bus Selector1/1
  Bus Selector1/1 -> Integrator/2  "<local_V_0>"
  [Initial_Conditions] -> Bus Selector2/1
  Bus Selector2/1 -> Unit Delay External IC/2  "<euler_0>"
  [Initial_Conditions] -> Bus Selector3/1
  Bus Selector3/1 -> Unit Delay External IC1/2  "<euler_0>"
  Bus Selector3/2 -> Unit Delay External IC2/2  "<alpha_0>"
  Bus Selector3/3 -> Unit Delay External IC3/2  "<beta_0>"
  [Initial_Conditions] -> Bus Selector4/1
  Bus Selector4/1 -> Unit Delay External IC4/2  "<airspeed_0>"
  Posicion MotorLeft/1 -> 3x3 Cross Product1/1
  3x3 Cross Product1/1 -> netsum5/3
  3x3 Cross Product2/1 -> netsum5/4
  Posicion MotorRight/1 -> 3x3 Cross Product2/1
  Control Surface Deflections/1 -> Subsystem/1(Control Surface Deflections)
  Motor stick position/1 -> Subsystem/2(Motor stick position)
  [Euler] -> Subsystem/3(Euler)
  netsum5/1 -> aceleraciones_angulares/1(M)
  Ecuaciones_de_Navegacion2/1(Mm) -> netsum5/1
  Ecuaciones_de_Navegacion1/1(Mm) -> netsum5/2
  Demux/2 -> Ecuaciones_de_Navegacion1/1(input)
  Demux/1 -> Ecuaciones_de_Navegacion2/1(input)
  Motor stick position1/1 -> Demux/1
  [MotorLeft] -> 3x3 Cross Product1/2
  [MotorRight] -> 3x3 Cross Product2/2
  Mux1/1 -> Global Velocities/1

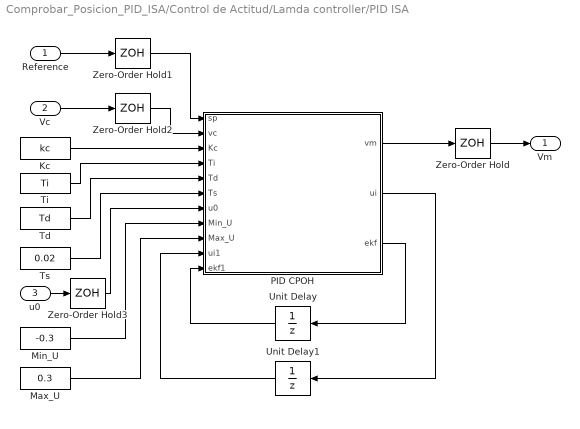
== system Comprobar_Posicion_PID_ISA/Control de Actitud/Lamda controller/PID ISA ==
  Reference : Inport
  Vc : Inport  Port=2
  u0 : Inport  Port=3
  Kc : Constant  Value=kc
  Max_U : Constant  Value=0.3
  Min_U : Constant  Value=-0.3
  PID CPOH : MATLAB Function  TreatAsAtomicUnit=on
  Td : Constant  Value=Td
  Ti : Constant  Value=Ti
  Ts : Constant  Value=0.02
  Unit Delay : UnitDelay  SampleTime=0.02  HasFrameUpgradeWarning=on
  Unit Delay1 : UnitDelay  SampleTime=0.02  HasFrameUpgradeWarning=on
  Zero-Order Hold : ZeroOrderHold  SampleTime=0.02
  Zero-Order Hold1 : ZeroOrderHold  SampleTime=0.02
  Zero-Order Hold2 : ZeroOrderHold  SampleTime=0.02
  Zero-Order Hold3 : ZeroOrderHold  SampleTime=0.04
  Vm : Outport
  wires:
  Kc/1 -> PID CPOH/3(Kc)
  Ti/1 -> PID CPOH/4(Ti)
  Td/1 -> PID CPOH/5(Td)
  Ts/1 -> PID CPOH/6(Ts)
  u0/1 -> Zero-Order Hold3/1
  Min_U/1 -> PID CPOH/8(Min_U)
  Max_U/1 -> PID CPOH/9(Max_U)
  Unit Delay/1 -> PID CPOH/11(ekf1)
  PID CPOH/3(ekf) -> Unit Delay/1
  Unit Delay1/1 -> PID CPOH/10(ui1)
  PID CPOH/2(ui) -> Unit Delay1/1
  Reference/1 -> Zero-Order Hold1/1
  Vc/1 -> Zero-Order Hold2/1
  PID CPOH/1(vm) -> Zero-Order Hold/1
  Zero-Order Hold/1 -> Vm/1
  Zero-Order Hold1/1 -> PID CPOH/1(sp)
  Zero-Order Hold3/1 -> PID CPOH/7(u0)
  Zero-Order Hold2/1 -> PID CPOH/2(vc)

== system Comprobar_Posicion_PID_ISA/Control de Actitud/Lamda controller/PID ISA1 ==
  Reference : Inport
  Vc : Inport  Port=2
  u0 : Inport  Port=3
  Kc : Constant  Value=kc
  Max_U : Constant  Value=0.4
  Min_U : Constant  Value=-0.4
  PID CPOH : MATLAB Function  TreatAsAtomicUnit=on
  Td : Constant  Value=Td
  Ti : Constant  Value=Ti
  Ts : Constant  Value=0.02
  Unit Delay : UnitDelay  SampleTime=0.02  HasFrameUpgradeWarning=on
  Unit Delay1 : UnitDelay  SampleTime=0.02  HasFrameUpgradeWarning=on
  Zero-Order Hold : ZeroOrderHold  SampleTime=0.02
  Zero-Order Hold1 : ZeroOrderHold  SampleTime=0.02
  Zero-Order Hold2 : ZeroOrderHold  SampleTime=0.02
  Zero-Order Hold3 : ZeroOrderHold  SampleTime=0.04
  Vm : Outport
  wires:
  Zero-Order Hold2/1 -> PID CPOH/2(vc)
  Zero-Order Hold3/1 -> PID CPOH/7(u0)
  Zero-Order Hold1/1 -> PID CPOH/1(sp)
  Zero-Order Hold/1 -> Vm/1
  PID CPOH/1(vm) -> Zero-Order Hold/1
  Vc/1 -> Zero-Order Hold2/1
  Reference/1 -> Zero-Order Hold1/1
  PID CPOH/2(ui) -> Unit Delay1/1
  Unit Delay1/1 -> PID CPOH/10(ui1)
  PID CPOH/3(ekf) -> Unit Delay/1
  Unit Delay/1 -> PID CPOH/11(ekf1)
  Max_U/1 -> PID CPOH/9(Max_U)
  Min_U/1 -> PID CPOH/8(Min_U)
  u0/1 -> Zero-Order Hold3/1
  Ts/1 -> PID CPOH/6(Ts)
  Td/1 -> PID CPOH/5(Td)
  Ti/1 -> PID CPOH/4(Ti)
  Kc/1 -> PID CPOH/3(Kc)

== system Comprobar_Posicion_PID_ISA/Control de Actitud/Thrust controller/PID ISA ==
  Reference : Inport
  Vc : Inport  Port=2
  u0 : Inport  Port=3
  Kc : Constant  Value=kc
  Max_U : Constant  Value=0.8
  Min_U : Constant  Value=0
  PID CPOH : MATLAB Function  TreatAsAtomicUnit=on
  Td : Constant  Value=Td
  Ti : Constant  Value=Ti
  Ts : Constant  Value=0.02
  Unit Delay : UnitDelay  SampleTime=0.02  HasFrameUpgradeWarning=on
  Unit Delay1 : UnitDelay  SampleTime=0.02  HasFrameUpgradeWarning=on
  Zero-Order Hold : ZeroOrderHold  SampleTime=0.02
  Zero-Order Hold1 : ZeroOrderHold  SampleTime=0.02
  Zero-Order Hold2 : ZeroOrderHold  SampleTime=0.02
  Zero-Order Hold3 : ZeroOrderHold  SampleTime=0.04
  Vm : Outport
  wires:
  Zero-Order Hold2/1 -> PID CPOH/2(vc)
  Zero-Order Hold3/1 -> PID CPOH/7(u0)
  Zero-Order Hold1/1 -> PID CPOH/1(sp)
  Zero-Order Hold/1 -> Vm/1
  PID CPOH/1(vm) -> Zero-Order Hold/1
  Vc/1 -> Zero-Order Hold2/1
  Reference/1 -> Zero-Order Hold1/1
  PID CPOH/2(ui) -> Unit Delay1/1
  Unit Delay1/1 -> PID CPOH/10(ui1)
  PID CPOH/3(ekf) -> Unit Delay/1
  Unit Delay/1 -> PID CPOH/11(ekf1)
  Max_U/1 -> PID CPOH/9(Max_U)
  Min_U/1 -> PID CPOH/8(Min_U)
  u0/1 -> Zero-Order Hold3/1
  Ts/1 -> PID CPOH/6(Ts)
  Td/1 -> PID CPOH/5(Td)
  Ti/1 -> PID CPOH/4(Ti)
  Kc/1 -> PID CPOH/3(Kc)

== system Comprobar_Posicion_PID_ISA/Control de Actitud/Thrust controller/PID ISA1 ==
  Reference : Inport
  Vc : Inport  Port=2
  u0 : Inport  Port=3
  Kc : Constant  Value=kc
  Max_U : Constant  Value=0.3
  Min_U : Constant  Value=-0.3
  PID CPOH : MATLAB Function  TreatAsAtomicUnit=on
  Td : Constant  Value=Td
  Ti : Constant  Value=Ti
  Ts : Constant  Value=0.02
  Unit Delay : UnitDelay  SampleTime=0.02  HasFrameUpgradeWarning=on
  Unit Delay1 : UnitDelay  SampleTime=0.02  HasFrameUpgradeWarning=on
  Zero-Order Hold : ZeroOrderHold  SampleTime=0.02
  Zero-Order Hold1 : ZeroOrderHold  SampleTime=0.02
  Zero-Order Hold2 : ZeroOrderHold  SampleTime=0.02
  Zero-Order Hold3 : ZeroOrderHold  SampleTime=0.04
  Vm : Outport
  wires:
  Kc/1 -> PID CPOH/3(Kc)
  Ti/1 -> PID CPOH/4(Ti)
  Td/1 -> PID CPOH/5(Td)
  Ts/1 -> PID CPOH/6(Ts)
  u0/1 -> Zero-Order Hold3/1
  Min_U/1 -> PID CPOH/8(Min_U)
  Max_U/1 -> PID CPOH/9(Max_U)
  Unit Delay/1 -> PID CPOH/11(ekf1)
  PID CPOH/3(ekf) -> Unit Delay/1
  Unit Delay1/1 -> PID CPOH/10(ui1)
  PID CPOH/2(ui) -> Unit Delay1/1
  Reference/1 -> Zero-Order Hold1/1
  Vc/1 -> Zero-Order Hold2/1
  PID CPOH/1(vm) -> Zero-Order Hold/1
  Zero-Order Hold/1 -> Vm/1
  Zero-Order Hold1/1 -> PID CPOH/1(sp)
  Zero-Order Hold3/1 -> PID CPOH/7(u0)
  Zero-Order Hold2/1 -> PID CPOH/2(vc)

== system Comprobar_Posicion_PID_ISA/Control de Actitud/Dynamic Model/VSkye/Euler_from_quaternions ==
  p q r : Inport
  Euler 0 : Constant  Value=euler_0
  Gain : Gain  Gain=0.5
  Integrator2 : Integrator  InitialConditionSource=external  InitialCondition=[0 0 0 0]  UpperSaturationLimit=Inf  LowerSaturationLimit=-Inf
  Memory : Memory  InitialCondition=[1 0 0 0]
  Mux : Mux  Inputs=2
  Quat scalar : Constant  Value=0
  Quaternion Multiplication : aerolibutil/Quaternion Multiplication
  Quaternions to Rotation Angles : sharedtransform/Quaternions to Rotation Angles  rotationOrder=ZYX  aMode=aMode
      settings: SourceProductBaseCode=AE,PW,DR,MT,UV,VE
  Rotation Angles to Quaternions : sharedtransform/Rotation Angles to Quaternions  rotationOrder=ZYX  aMode=aMode
      settings: SourceProductBaseCode=AE,PW,DR,MT,UV,VE
  Selector2 : Selector  InputPortWidth=3  IndexOptions=Index vector (dialog)  Indices=[3 2 1]  OutputSizes=1
  Euler : Outport
  wires:
  Quaternion Multiplication/1 -> Integrator2/1  "quaternionDot"
  Rotation Angles to Quaternions/1 -> Integrator2/2
  Integrator2/1 -> Quaternions to Rotation Angles/1, Memory/1
  Mux/1 -> Gain/1
  Gain/1 -> Quaternion Multiplication/1
  Memory/1 -> Quaternion Multiplication/2
  Quat scalar/1 -> Mux/1
  p q r/1 -> Selector2/1
  Euler 0/1 -> Rotation Angles to Quaternions/1
  Quaternions to Rotation Angles/1 -> Euler/1
  Selector2/1 -> Mux/2

== system Comprobar_Posicion_PID_ISA/Control de Actitud/Dynamic Model/VSkye/Initial_Conditions ==
  Bus Creator : BusCreator  Inputs=13
  Embedded MATLAB Function : MATLAB Function  TreatAsAtomicUnit=on
  Gain : Gain  Gain=-1
  Pos_0 : Constant  Value=Pos_0
  Vel_0 : Constant  Value=Vel_0
  airspeed_0 : Constant  Value=airspeed_0
  alpha_0 : Constant  Value=alpha_0
  altitude_0 : Constant  Value=altitude_0
  beta_0 : Constant  Value=beta_0
  deflect_sat : Constant  Value=deflect_sat
  euler_0 : Constant  Value=euler_0
  h0 : Constant  Value=h0
  local_V_0 : Constant  Value=local_V_0
  pqr_0 : Constant  Value=pqr_0
  theta_0 : Constant  Value=theta_0
  Initial_Conditions : Outport
  wires:
  Bus Creator/1 -> Initial_Conditions/1
  Vel_0/1 -> Bus Creator/1, Embedded MATLAB Function/1(Vel_0)  "Vel_0"
  Pos_0/1 -> Bus Creator/2  "Pos_0"
  h0/1 -> Bus Creator/3  "h0"
  Embedded MATLAB Function/1(V_air_0) -> Bus Creator/4  "V_air_0"
  pqr_0/1 -> Bus Creator/5  "pqr_0"
  euler_0/1 -> Bus Creator/6  "euler_0"
  theta_0/1 -> Bus Creator/7  "theta_0"
  deflect_sat/1 -> Bus Creator/8  "deflect_sat"
  alpha_0/1 -> Bus Creator/9  "alpha_0"
  beta_0/1 -> Bus Creator/10  "beta_0"
  local_V_0/1 -> Bus Creator/11  "local_V_0"
  altitude_0/1 -> Gain/1  "altitude_0"
  Gain/1 -> Bus Creator/12  "altitude_0"
  airspeed_0/1 -> Bus Creator/13  "airspeed_0"

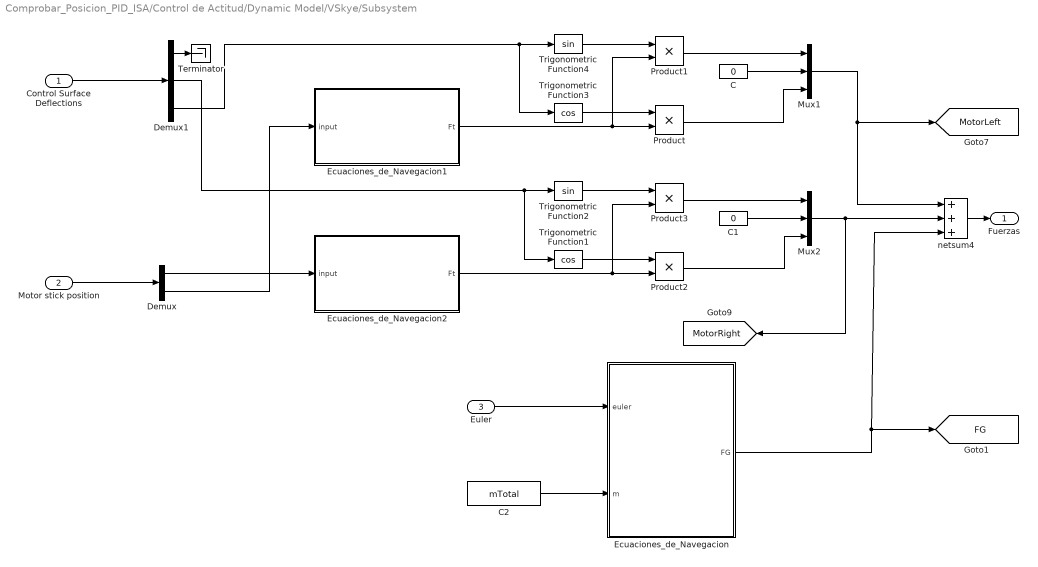
== system Comprobar_Posicion_PID_ISA/Control de Actitud/Dynamic Model/VSkye/Subsystem ==
  Control Surface Deflections : Inport
  Motor stick position : Inport  Port=2
  Euler : Inport  Port=3
  "C " : Constant  Value=0
  C1 : Constant  Value=0
  C2 : Constant  Value=mTotal
  Demux : Demux  Outputs=2
  Demux1 : Demux  Outputs=3
  Ecuaciones_de_Navegacion : MATLAB Function  TreatAsAtomicUnit=on
  Ecuaciones_de_Navegacion1 : MATLAB Function  TreatAsAtomicUnit=on
  Ecuaciones_de_Navegacion2 : MATLAB Function  TreatAsAtomicUnit=on
  Mux1 : Mux  Inputs=3
  Mux2 : Mux  Inputs=3
  Product{,1..3} (4 alike) : Product  RndMeth=Zero
  Terminator : Terminator
  Trigonometric Function1 : Trigonometry  Operator=cos
  Trigonometric Function2 : Trigonometry
  Trigonometric Function3 : Trigonometry  Operator=cos
  Trigonometric Function4 : Trigonometry
  netsum4 : Sum  Inputs=3  InputSameDT=on  SaturateOnIntegerOverflow=on  OutDataTypeStr=Inherit: Same as first input
  Fuerzas : Outport
  tag scope: FG=global, MotorLeft=global, MotorRight=global
  wires:
  "C "/1 -> Mux1/2
  C1/1 -> Mux2/2
  Ecuaciones_de_Navegacion/1(FG) -> netsum4/3, [FG]
  C2/1 -> Ecuaciones_de_Navegacion/2(m)
  Demux/2 -> Ecuaciones_de_Navegacion1/1(input)
  Demux1/3 -> Trigonometric Function4/1, Trigonometric Function3/1
  Product/1 -> Mux1/3
  Ecuaciones_de_Navegacion1/1(Ft) -> Product1/2, Product/2
  Trigonometric Function3/1 -> Product/1
  Trigonometric Function4/1 -> Product1/1
  Product1/1 -> Mux1/1
  Demux1/2 -> Trigonometric Function2/1, Trigonometric Function1/1
  Ecuaciones_de_Navegacion2/1(Ft) -> Product3/2, Product2/2
  Trigonometric Function1/1 -> Product2/1
  Trigonometric Function2/1 -> Product3/1
  Product2/1 -> Mux2/3
  Product3/1 -> Mux2/1
  Motor stick position/1 -> Demux/1
  Control Surface Deflections/1 -> Demux1/1
  netsum4/1 -> Fuerzas/1
  Euler/1 -> Ecuaciones_de_Navegacion/1(euler)
  Demux1/1 -> Terminator/1
  Demux/1 -> Ecuaciones_de_Navegacion2/1(input)
  Mux1/1 -> [MotorLeft], netsum4/1
  Mux2/1 -> [MotorRight], netsum4/2

== matlab function Comprobar_Posicion_PID_ISA/Control de Actitud/Thrust controller/PID ISA/PID CPOH ==
  data: sp input; vm output; vc input; Kc input; Ti input; Td input; Ts input; u0 input; Min_U input; Max_U input; ui1 input; ekf1 input; ui output; ekf output
function [vm,ui,ekf] = fcn(sp,vc,Kc,Ti,Td,Ts,u0,Min_U,Max_U,ui1,ekf1)

% Variables auxiliares...
N =0;         % N=0 desconecta el filtro de la derivada
b  = 1;       % Ponderación de la ref en la acción Proporcional
c  = 1;       % Ponderación de la ref en la acción derivada
offset = u0;  % offset, incluye el efecto de los puntos de
ki = 0;

if (Ti~=0)
    ki = (Kc*Ts)/Ti;
end

kd = (Kc*Td)/Ts;

if N~=0
    kn =Td/(N*Ts);
end

tauf = 0;
kf = tauf/Ts;

% Filtrado de la medida
if tauf == 0
    ykf=vc;
else
    ykf=(kf*ykf1+vc)/(kf+1);
end

% cálculo termino proporcional...
% con ponderacion de la referencia...
up=Kc*(b*sp-ykf);

% cálculo del termino derivada...
% con ponderacion de la referencia...
% y filtrado...

if (Td==0)
    ud=0;
    ekf=0;
else
    ek=c*sp-ykf;
    if N==0
        ekf=ek;
    else
        ekf=(kn*ekf1+ek)/(kn+1);
    end
    ud=kd*(ekf-ekf1);
end

% cálculo termino integral...
if (Ti==0)
    ui=0;
else
    ui=ui1+ki*(sp-ykf);
end
vm = up+ui+ud+offset;

% Antiwindup...
% saturación del incremento mínimo (El incremento mínimo es de 0.005 mm)
% saturación de la acción de control.
if (vm < Min_U)
    ui=ui1;
    vm=Min_U;
end
if (vm > Max_U)
    ui=ui1;
    vm= Max_U;
end

== matlab function Comprobar_Posicion_PID_ISA/Control de Actitud/Lamda controller/PID ISA/PID CPOH ==
  data: sp input; vm output; vc input; Kc input; Ti input; Td input; Ts input; u0 input; Min_U input; Max_U input; ui1 input; ekf1 input; ui output; ekf output
function [vm,ui,ekf] = fcn(sp,vc,Kc,Ti,Td,Ts,u0,Min_U,Max_U,ui1,ekf1)

% Variables auxiliares...
N =0;         % N=0 desconecta el filtro de la derivada
b  = 1;       % Ponderación de la ref en la acción Proporcional
c  = 1;       % Ponderación de la ref en la acción derivada
offset = u0;  % offset, incluye el efecto de los puntos de
ki = 0;

if (Ti~=0)
    ki = (Kc*Ts)/Ti;
end

kd = (Kc*Td)/Ts;

if N~=0
    kn =Td/(N*Ts);
end

tauf = 0;
kf = tauf/Ts;

% Filtrado de la medida
if tauf == 0
    ykf=vc;
else
    ykf=(kf*ykf1+vc)/(kf+1);
end

% cálculo termino proporcional...
% con ponderacion de la referencia...
up=Kc*(b*sp-ykf);

% cálculo del termino derivada...
% con ponderacion de la referencia...
% y filtrado...

if (Td==0)
    ud=0;
    ekf=0;
else
    ek=c*sp-ykf;
    if N==0
        ekf=ek;
    else
        ekf=(kn*ekf1+ek)/(kn+1);
    end
    ud=kd*(ekf-ekf1);
end

% cálculo termino integral...
if (Ti==0)
    ui=0;
else
    ui=ui1+ki*(sp-ykf);
end
vm = up+ui+ud+offset;

% Antiwindup...
% saturación del incremento mínimo (El incremento mínimo es de 0.005 mm)
% saturación de la acción de control.
if (vm < Min_U)
    ui=ui1;
    vm=Min_U;
end
if (vm > Max_U)
    ui=ui1;
    vm= Max_U;
end

== matlab function Comprobar_Posicion_PID_ISA/Control de Actitud/Thrust controller/PID ISA1/PID CPOH ==
  data: sp input; vm output; vc input; Kc input; Ti input; Td input; Ts input; u0 input; Min_U input; Max_U input; ui1 input; ekf1 input; ui output; ekf output
function [vm,ui,ekf] = fcn(sp,vc,Kc,Ti,Td,Ts,u0,Min_U,Max_U,ui1,ekf1)

% Variables auxiliares...
N =0;         % N=0 desconecta el filtro de la derivada
b  = 1;       % Ponderación de la ref en la acción Proporcional
c  = 1;       % Ponderación de la ref en la acción derivada
offset = u0;  % offset, incluye el efecto de los puntos de
ki = 0;

if (Ti~=0)
    ki = (Kc*Ts)/Ti;
end

kd = (Kc*Td)/Ts;

if N~=0
    kn =Td/(N*Ts);
end

tauf = 0;
kf = tauf/Ts;

% Filtrado de la medida
if tauf == 0
    ykf=vc;
else
    ykf=(kf*ykf1+vc)/(kf+1);
end

% cálculo termino proporcional...
% con ponderacion de la referencia...
up=Kc*(b*sp-ykf);

% cálculo del termino derivada...
% con ponderacion de la referencia...
% y filtrado...

if (Td==0)
    ud=0;
    ekf=0;
else
    ek=c*sp-ykf;
    if N==0
        ekf=ek;
    else
        ekf=(kn*ekf1+ek)/(kn+1);
    end
    ud=kd*(ekf-ekf1);
end

% cálculo termino integral...
if (Ti==0)
    ui=0;
else
    ui=ui1+ki*(sp-ykf);
end
vm = up+ui+ud+offset;

% Antiwindup...
% saturación del incremento mínimo (El incremento mínimo es de 0.005 mm)
% saturación de la acción de control.
if (vm < Min_U)
    ui=ui1;
    vm=Min_U;
end
if (vm > Max_U)
    ui=ui1;
    vm= Max_U;
end

== matlab function Comprobar_Posicion_PID_ISA/posz controller1/PID ISA/PID CPOH ==
  data: sp input; vm output; vc input; Kc input; Ti input; Td input; Ts input; u0 input; Min_U input; Max_U input; ui1 input; ekf1 input; ui output; ekf output
function [vm,ui,ekf] = fcn(sp,vc,Kc,Ti,Td,Ts,u0,Min_U,Max_U,ui1,ekf1)

% Variables auxiliares...
N =0;         % N=0 desconecta el filtro de la derivada
b  = 1;       % Ponderación de la ref en la acción Proporcional
c  = 1;       % Ponderación de la ref en la acción derivada
offset = u0;  % offset, incluye el efecto de los puntos de
ki = 0;

if (Ti~=0)
    ki = (Kc*Ts)/Ti;
end

kd = (Kc*Td)/Ts;

if N~=0
    kn =Td/(N*Ts);
end

tauf = 0;
kf = tauf/Ts;

% Filtrado de la medida
if tauf == 0
    ykf=vc;
else
    ykf=(kf*ykf1+vc)/(kf+1);
end

% cálculo termino proporcional...
% con ponderacion de la referencia...
up=Kc*(b*sp-ykf);

% cálculo del termino derivada...
% con ponderacion de la referencia...
% y filtrado...

if (Td==0)
    ud=0;
    ekf=0;
else
    ek=c*sp-ykf;
    if N==0
        ekf=ek;
    else
        ekf=(kn*ekf1+ek)/(kn+1);
    end
    ud=kd*(ekf-ekf1);
end

% cálculo termino integral...
if (Ti==0)
    ui=0;
else
    ui=ui1+ki*(sp-ykf);
end
vm = up+ui+ud+offset;

% Antiwindup...
% saturación del incremento mínimo (El incremento mínimo es de 0.005 mm)
% saturación de la acción de control.
if (vm < Min_U)
    ui=ui1;
    vm=Min_U;
end
if (vm > Max_U)
    ui=ui1;
    vm= Max_U;
end

== matlab function Comprobar_Posicion_PID_ISA/posy controller1/PID ISA/PID CPOH ==
  data: sp input; vm output; vc input; Kc input; Ti input; Td input; Ts input; u0 input; Min_U input; Max_U input; ui1 input; ekf1 input; ui output; ekf output
function [vm,ui,ekf] = fcn(sp,vc,Kc,Ti,Td,Ts,u0,Min_U,Max_U,ui1,ekf1)

% Variables auxiliares...
N =0;         % N=0 desconecta el filtro de la derivada
b  = 1;       % Ponderación de la ref en la acción Proporcional
c  = 1;       % Ponderación de la ref en la acción derivada
offset = u0;  % offset, incluye el efecto de los puntos de
ki = 0;

if (Ti~=0)
    ki = (Kc*Ts)/Ti;
end

kd = (Kc*Td)/Ts;

if N~=0
    kn =Td/(N*Ts);
end

tauf = 0;
kf = tauf/Ts;

% Filtrado de la medida
if tauf == 0
    ykf=vc;
else
    ykf=(kf*ykf1+vc)/(kf+1);
end

% cálculo termino proporcional...
% con ponderacion de la referencia...
up=Kc*(b*sp-ykf);

% cálculo del termino derivada...
% con ponderacion de la referencia...
% y filtrado...

if (Td==0)
    ud=0;
    ekf=0;
else
    ek=c*sp-ykf;
    if N==0
        ekf=ek;
    else
        ekf=(kn*ekf1+ek)/(kn+1);
    end
    ud=kd*(ekf-ekf1);
end

% cálculo termino integral...
if (Ti==0)
    ui=0;
else
    ui=ui1+ki*(sp-ykf);
end
vm = up+ui+ud+offset;

% Antiwindup...
% saturación del incremento mínimo (El incremento mínimo es de 0.005 mm)
% saturación de la acción de control.
if (vm < Min_U)
    ui=ui1;
    vm=Min_U;
end
if (vm > Max_U)
    ui=ui1;
    vm= Max_U;
end

== matlab function Comprobar_Posicion_PID_ISA/Control de Actitud/Dynamic Model/VSkye/Subsystem/Ecuaciones_de_Navegacion ==
  data: FG output; euler input; m input
function FG = F_gravedad(euler,m)
g=9.81;
FG=m*g*[-sin(euler(2));sin(euler(1))*cos(euler(2));cos(euler(1))*cos(euler(2))];
end

== matlab function Comprobar_Posicion_PID_ISA/posx controller1/PID ISA/PID CPOH ==
  data: sp input; vm output; vc input; Kc input; Ti input; Td input; Ts input; u0 input; Min_U input; Max_U input; ui1 input; ekf1 input; ui output; ekf output
function [vm,ui,ekf] = fcn(sp,vc,Kc,Ti,Td,Ts,u0,Min_U,Max_U,ui1,ekf1)

% Variables auxiliares...
N =0;         % N=0 desconecta el filtro de la derivada
b  = 1;       % Ponderación de la ref en la acción Proporcional
c  = 1;       % Ponderación de la ref en la acción derivada
offset = u0;  % offset, incluye el efecto de los puntos de
ki = 0;

if (Ti~=0)
    ki = (Kc*Ts)/Ti;
end

kd = (Kc*Td)/Ts;

if N~=0
    kn =Td/(N*Ts);
end

tauf = 0;
kf = tauf/Ts;

% Filtrado de la medida
if tauf == 0
    ykf=vc;
else
    ykf=(kf*ykf1+vc)/(kf+1);
end

% cálculo termino proporcional...
% con ponderacion de la referencia...
up=Kc*(b*sp-ykf);

% cálculo del termino derivada...
% con ponderacion de la referencia...
% y filtrado...

if (Td==0)
    ud=0;
    ekf=0;
else
    ek=c*sp-ykf;
    if N==0
        ekf=ek;
    else
        ekf=(kn*ekf1+ek)/(kn+1);
    end
    ud=kd*(ekf-ekf1);
end

% cálculo termino integral...
if (Ti==0)
    ui=0;
else
    ui=ui1+ki*(sp-ykf);
end
vm = up+ui+ud+offset;

% Antiwindup...
% saturación del incremento mínimo (El incremento mínimo es de 0.005 mm)
% saturación de la acción de control.
if (vm < Min_U)
    ui=ui1;
    vm=Min_U;
end
if (vm > Max_U)
    ui=ui1;
    vm= Max_U;
end

== matlab function Comprobar_Posicion_PID_ISA/Control de Actitud/Dynamic Model/VSkye/Initial_Conditions/Embedded MATLAB Function ==
  data: Vel_0 input; V_air_0 output
function V_air_0 = fcn(Vel_0)
%#eml

V_air_0=sqrt(Vel_0(1)^2 + Vel_0(2)^2 + Vel_0(1)^2);

== matlab function Comprobar_Posicion_PID_ISA/Control de Actitud/Dynamic Model/VSkye/Subsystem/Ecuaciones_de_Navegacion1 ==
  data: Ft output; input input
function Ft=fuerza_Motor(input)
%g=9.81;
%Ft=(1/3.27193530612245)*(-0.0292*(input*100).^2 + 36.681*(input*100) - 107.5)*g/1000;%en N;
Ft=-9.8*input;

end

== matlab function Comprobar_Posicion_PID_ISA/Control de Actitud/Dynamic Model/VSkye/Subsystem/Ecuaciones_de_Navegacion2 ==
  data: Ft output; input input
function Ft=fuerza_Motor(input)
%g=9.81;
%Ft=(1/3.27193530612245)*(-0.0292*(input*100).^2 + 36.681*(input*100) - 107.5)*g/1000;%en N;
Ft=-9.8*input;
end

== matlab function Comprobar_Posicion_PID_ISA/Control de Actitud/Dynamic Model/VSkye/Wind variables ==
  data: V_vector input; euler input; alpha output; beta output; air_uvw output; W_vector input; airspeed output
function [alpha , beta, air_uvw ,airspeed] = fcn(V_vector, euler ,W_vector)

% Wx=W_vector(1);
% Wy=W_vector(2);
% Wz=W_vector(3);

roll=euler(1);
pitch=euler(2);
yaw=euler(3);

Cx=[[1 0 0];[0 cos(roll) sin(roll)];[0 -sin(roll) cos(roll)]];
Cy=[[cos(pitch) 0 -sin(pitch)];[0 1 0];[sin(pitch) 0 cos(pitch)]];
Cz=[[cos(yaw) sin(yaw) 0];[-sin(yaw) cos(yaw) 0];[0 0 1]];

W_vector_local=(Cx*Cy*Cz)*W_vector;

airspeed_vector=V_vector-W_vector_local;

u=airspeed_vector(1);
v=airspeed_vector(2);
w=airspeed_vector(3);

air_uvw=[u;v;w];

airspeed=sqrt(u^2+v^2+w^2);

alpha = atan2(w,u);
beta  = asin(v/airspeed);

end

== matlab function Comprobar_Posicion_PID_ISA/Control de Actitud/Dynamic Model/VSkye/Ecuaciones_de_Navegacion2 ==
  data: Mm output size=3; input input
function Mm=par_Motor(input)
%g=9.81;
C_P=0.04;
C_T=0.08;
INCH2M=2.54e-2;
D=8*INCH2M;
Kpar=D*C_P/(2*pi()*C_T);
%Ft=(1/3.27193530612245)*(-0.0292*(input*100).^2 + 36.681*(input*100) - 107.5)*g/1000;%en N;
Ft=-9.8*input;
Par=Kpar*Ft;%en Nm;

Mm=[0;0;Par];
end

== matlab function Comprobar_Posicion_PID_ISA/Control de Actitud/Dynamic Model/VSkye/aceleraciones_angulares ==
  data: M input; vel_ang input; acc_ang output
function acc_ang = aceleraciones_ang(M,vel_ang)

    Ix=0.049881949093749;
    Iy=0.016478266864509;
    Iz=0.033418277170000;
    Ixz=4.708766122801070e-06;

    
    A_aux=[[1 -Ixz/Ix];[-Ixz/Iz 1]];
    B_aux=[(M(1) - vel_ang(2)*vel_ang(3)*(Iz-Iy)...
                 + vel_ang(2)*vel_ang(1)*Ixz)/Ix;...

           (M(3) - vel_ang(1)*vel_ang(2)*(Iy-Ix)...
                 - vel_ang(2)*vel_ang(3)*Ixz)/Iz];

    aux=(A_aux^(-1))*B_aux;


    p_dot=aux(1);

    q_dot=(M(2)-vel_ang(1)*vel_ang(3)*(Ix-Iz)...
          -(vel_ang(1)^2-vel_ang(3)^2)*Ixz)/Iy;

    r_dot=aux(2);

    acc_ang=[p_dot;q_dot;r_dot];
    
end
